simulink model "MotorModelVariableOld"  (R2015b)
settings: Solver=VariableStepAuto  StartTime=0.0  StopTime=10.0  RelTol=1e-3
undefined symbols (not defined in the file): Initial, Motor, Uav
libraries: simulink_extras x1
settings Model: Creator=jban039  LastModifiedBy=jban039

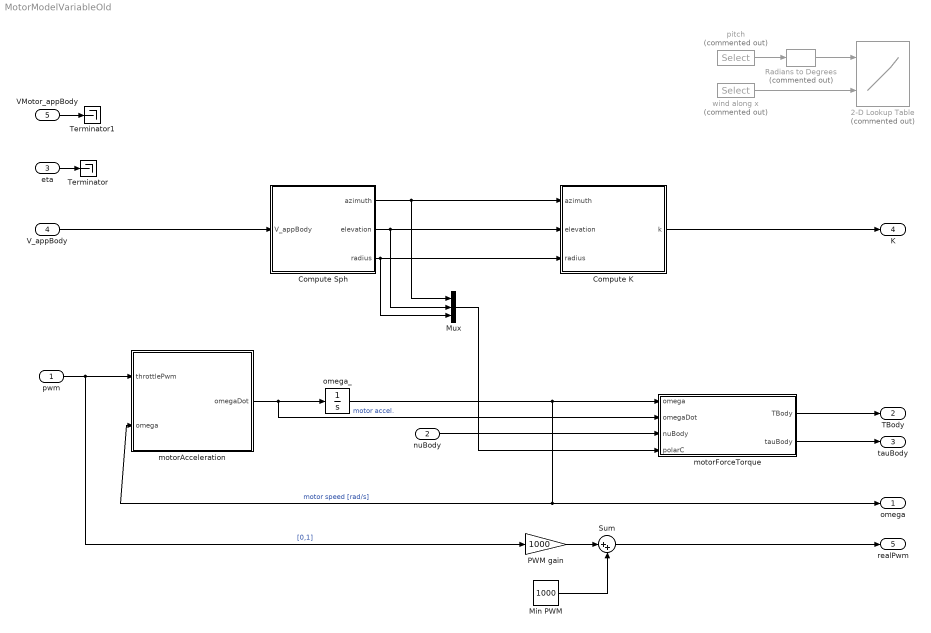
== system MotorModelVariableOld ==
  pwm : Inport  PortDimensions=Uav.N_ROTORS
  nuBody : Inport  Port=2
  eta : Inport  Port=3  PortDimensions=3
  V_appBody : Inport  Port=4  PortDimensions=3
  VMotor_appBody : Inport  Port=5  PortDimensions=[3,4]
  2-D Lookup Table : Lookup_n-D  Commented=on  BreakpointsForDimension1=[0,2.890909,6.009259676377,9.296238414,12.27875]  BreakpointsForDimension2=[0,10,20]  Table=reshape([9.55641004221352e-06,1.00990801427108e-05,1.28091919414946e-05,1.45562427543497e-05,1.63017404112369e-05,1.00884339028815e-05,1.06718323589317e-05,1.12577089455794e-05,1.21229824131359e-05,1.24606394544993e-05,9.47230336229989e-06,9.71233115660863e-06,9.65341998978562e-06,9.60249125674676e-06,8.92828582195144e-06],5,3)  InternalRulePriority=Speed  RndMeth=Simplest  InputSameDT=on
  Compute K : MATLAB Function  TreatAsAtomicUnit=on
  Compute Sph : MATLAB Function  TreatAsAtomicUnit=on
  Min PWM : Constant  Value=1000
  Mux : Mux  Inputs=3
  PWM gain : Gain  Gain=1000
  Radians to Degrees : simulink_extras/Transformations/Radians to Degrees  Commented=on
  Sum : Sum  Inputs=|++
  Terminator : Terminator
  Terminator1 : Terminator
  motorAcceleration : MATLAB Function  TreatAsAtomicUnit=on
  motorForceTorque : MATLAB Function  TreatAsAtomicUnit=on
  omega_ : Integrator  InitialCondition=Initial.OMEGA
  pitch : Selector  Commented=on  InputPortWidth=3  IndexOptions=Index vector (dialog)  Indices=[2]  OutputSizes=1
  wind along x : Selector  Commented=on  InputPortWidth=3  IndexOptions=Index vector (dialog)  Indices=[1]  OutputSizes=1
  omega : Outport
  TBody : Outport  Port=2
  tauBody : Outport  Port=3
  K : Outport  Port=4
  realPwm : Outport  Port=5
  wires:
  motorAcceleration/1(omegaDot) -> motorForceTorque/2(omegaDot), omega_/1  "motor accel."
  motorForceTorque/2(tauBody) -> tauBody/1
  motorForceTorque/1(TBody) -> TBody/1
  omega_/1 -> motorAcceleration/2(omega), omega/1, motorForceTorque/1(omega)  "motor speed [rad/s]"
  nuBody/1 -> motorForceTorque/3(nuBody)
  wind along x/1 -> 2-D Lookup Table/2
  pitch/1 -> Radians to Degrees/1
  Compute K/1(k) -> K/1
  Radians to Degrees/1 -> 2-D Lookup Table/1
  eta/1 -> Terminator/1
  V_appBody/1 -> Compute Sph/1(V_appBody)
  Compute Sph/3(radius) -> Mux/3, Compute K/3(radius)
  Compute Sph/1(azimuth) -> Mux/1, Compute K/1(azimuth)
  Compute Sph/2(elevation) -> Mux/2, Compute K/2(elevation)
  Mux/1 -> motorForceTorque/4(polarC)
  pwm/1 -> PWM gain/1, motorAcceleration/1(throttlePwm)  "[0,1]"
  Sum/1 -> realPwm/1
  PWM gain/1 -> Sum/1
  Min PWM/1 -> Sum/2
  VMotor_appBody/1 -> Terminator1/1

== matlab function MotorModelVariableOld/Compute Sph ==
  data: V_appBody input; azimuth output; elevation output; radius output
function [azimuth, elevation, radius] = computeSph(V_appBody)
%#codegen

% Convert from polar to spherical coordinates
[ azimuth, elevation, radius ] = cart2sph( V_appBody(1), V_appBody(2), V_appBody(3) );

== matlab function MotorModelVariableOld/Compute K ==
  data: azimuth input; k output; elevation input; radius input
function k  = computeK( azimuth, elevation, radius )
%#codegen

% Margin to prevent shattering - doesn't seem to work
% for i = 1:3
%     if ( ( V_appBody(i) > -0.002 ) && ( V_appBody(i) < 0.002 ) )
%         V_appBody(i) = 0;
%     end
% end

% % Convert from polar to spherical coordinates
% [ azimuth, elevation, radius ] = cart2sph( V_appBody(1), V_appBody(2), V_appBody(3) );

elevation = abs(elevation);

if ( elevation < 0 )
    elevation = 0;
elseif ( elevation > pi/4 )
    elevation = pi/4;
end

% if ( ( elevation < 0 ) || ( radius < 0.02 ) ) %  || ( abs( azimuth ) > pi / 4 )
%     k = 9.20186997424055e-06;
% else
k =  9.20186997424055e-06 + ...
     4.85267548640599e-06 * elevation + ...
     5.76685430140641e-07 * radius  + ...
    -8.78213951736416e-06 * elevation .^ 2 +...
    -1.77642149547229e-06 * elevation * radius + ...
    -1.52971221787416e-09 * radius^2;

k = 7.59588e-6;

% if ( k < 9.20186997424055e-06 )
%     k = 9.20186997424055e-06;
% end
% end

== matlab function MotorModelVariableOld/motorForceTorque ==
  data: omega input; TBody output size=3; omegaDot input; nuBody input size=3; Motor parameter; Uav parameter; tauBody output size=3; polarC input
function [TBody, tauBody] = motorForceTorque(...
    omega, omegaDot, nuBody, Motor, Uav, polarC)
%#codegen

elevation = polarC(2);
windSpeed = polarC(3);

% Make assertions to avoid code generation errors
assert(Uav.N_ROTORS < 16);

%% Thrust and differential torque

% Concatenated motor force/torque vectors in respective motor frame
% eg. TMotor = [TMotor1, TMotor2, ..., TMotorN]
% where: - N is the number of rotors
%        - TMotorx (x ∈ [1,2,...,N]) is the thrust generated by motor x in
%          its own frame of reference
% TMotorIndividual = [ zeros(2, Uav.N_ROTORS);
%                      K * (omega'.^2) ];
K1 = 6.543988868292138e-05+...
    1.886359198743874e-06*sin(elevation)+...
    -7.693938774360465e-07*windSpeed+...
    2.639630950517221e-06*sin(elevation)*windSpeed+...
    2.126334444415667e-08*windSpeed^2;
K2 = -1.903771811601254e-04+...
    2.812570127999989e-03*sin(elevation)+...
    1.418616236881443e-03*windSpeed+...
    -4.525882966383329e-03*sin(elevation)*windSpeed+...
    -1.658875316836167e-05*windSpeed^2;
TMotorIndividual = [ zeros(2, Uav.N_ROTORS);
                     0.5 * Uav.RHO_AIR * K1 * (omega'.^2) + 0.5 * Uav.RHO_AIR * K2 * (omega') ];
tauMotorIndividual = [ zeros(2, Uav.N_ROTORS);
                      -Uav.ROTOR_DIRECTION .* ...
                 ( Motor.B*(omega'.^2) + Motor.I_R(3,3)*omegaDot' ) ];

% Initialise matrices to store motor force/torque vectors in body frame
TBodyIndividual   = zeros(3, Uav.N_ROTORS);
tauBodyIndividual = zeros(3, Uav.N_ROTORS);

% Calculate forces and moments from each motor in the body frame
for i = 1:Uav.N_ROTORS
    l = Uav.L(i);
    beta = Uav.BETA(i);
    
    % Matrix to compute torque applied by rotor thrust
 	L = [ 0,            0,            l*sin(beta);
          0,            0,           -l*cos(beta);
         -l*sin(beta),  l*cos(beta),  0 ];

	% Motor force/torque vectors in body frame
	TBodyIndividual(:,i) = Uav.R_MOTOR_TO_BODY(:,:,i) * ...
        TMotorIndividual(:,i);
	tauBodyIndividual(:,i) = Uav.R_MOTOR_TO_BODY(:,:,i) * ...
        tauMotorIndividual(:,i) + L * TBodyIndividual(:,i);
end

%% Gyroscopic moments

% Concatenated gyroscopic moments for each rotor
M_GBodyIndividual = zeros(3, Uav.N_ROTORS);

% Concatenated motor speeds in their respective frames
omegaMotor = [ zeros(2, Uav.N_ROTORS);
               Uav.ROTOR_DIRECTION .* omega' ];

% Angular momentum in motor frame
H_MMotorSeparate = Motor.I_R * omegaMotor;

% Gyroscopic moment vectors in body frame
for i = 1:Uav.N_ROTORS
	M_GBodyIndividual(:,i) = cross( nuBody, ...
        Uav.R_MOTOR_TO_BODY(:,:,i) * H_MMotorSeparate(:,i) );
end

M_GBody = sum(M_GBodyIndividual, 2);

%% Total torque and moment

% Total force/torque in body frame
TBody = sum(TBodyIndividual, 2);
tauBody = sum(tauBodyIndividual, 2) - M_GBody;

end

== matlab function MotorModelVariableOld/motorAcceleration ==
  data: throttlePwm input; omegaDot output double size=4; omega input; Motor parameter; Uav parameter
function omegaDot = motorAcceleration(throttlePwm, omega, Motor, Uav)
%#codegen

voltage = throttlePwm * Uav.NOMINAL_BATTERY_VOLTAGE;

% Motor current ignoring inductance
current = (voltage - Motor.K_E*omega) / Motor.R;

netTorque = (Motor.K_T * current) - (Motor.B * omega.^2);

% Motor angular acceleration
omegaDot = netTorque / Motor.I_R(3,3);
